simulink model "ExpCtrl"  (R2013a)
settings: Solver=ode45  StartTime=0.0  StopTime=10.0  RelTol=1e-3
libraries: mpt_sim x1
settings Model: Creator=root  LastModifiedBy=root

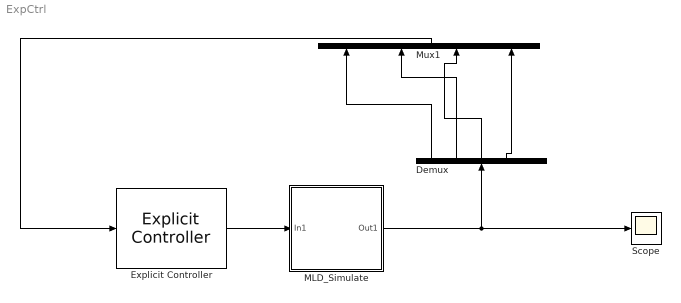
== system ExpCtrl ==
  Demux : Demux  Outputs=5
  Explicit Controller : mpt_sim/Explicit Controller
  MLD_Simulate : Subsystem
  Mux1 : Mux
  Scope : Scope
  wires:
  Explicit Controller/1 -> MLD_Simulate/1(In1)
  MLD_Simulate/1(Out1) -> Scope/1, Demux/1
  Demux/1 -> Mux1/1
  Demux/2 -> Mux1/2
  Demux/3 -> Mux1/3
  Demux/4 -> Mux1/4
  Mux1/1 -> Explicit Controller/1

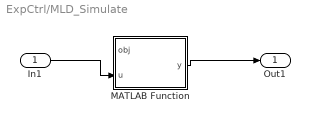
== system ExpCtrl/MLD_Simulate ==
  In1 : Inport
  MATLAB Function : MATLAB Function  TreatAsAtomicUnit=on
  Out1 : Outport
  wires:
  In1/1 -> MATLAB Function/2(u)
  MATLAB Function/1(y) -> Out1/1

== matlab function ExpCtrl/MLD_Simulate/MATLAB Function ==
  data: obj input; u input; y output
function y = fcn(obj,u)
%#codegen

y = obj.update(u);
